simulink model "UTSG11111"  (R2016a)
settings: Solver=VariableStepAuto  StartTime=0.0  StopTime=10.0  RelTol=1e-3
values from neighbouring files (symbols this model uses):
  A_dw = 110.74    [zmienne.m]
  A_fs = 60.67    [zmienne.m]
  A_p = (PI * (D_i^2) * N) / (4 * 144)    (= 11.0984259136)    [zmienne.m]
  C_1 = 1 / sqrt(C_d)    [zmienne.m]
  C_m = 0.11    [zmienne.m]
  C_p1 = 1.39    [zmienne.m]
  C_p2 = 1.165    [zmienne.m]
  DENS_d = 50.32    [zmienne.m]
  DENS_dw = 47.66    [zmienne.m]
  DENS_s = 52.32    [zmienne.m]
  DENS_w = 45.710    (= 45.71)    [zmienne.m]
  G_1 = 65.2    [zmienne.m]
  G_2 = 1.0    (= 1)    [zmienne.m]
  G_v = 32.2    [zmienne.m]
  K1 = 3.5 * 10^-6    (= 3.5e-06)    [zmienne.m]
  K2 = -7.135 * 10^-4    (= -0.0007135)    [zmienne.m]
  K3 = 0.17    [zmienne.m]
  K4 = -0.2    [zmienne.m]
  K5 = 0.14    [zmienne.m]
  K7 = 2.37 * 10^-3    (= 0.00237)    [zmienne.m]
  L = 35.54    [zmienne.m]
  L_d = 35.54    [zmienne.m]
  L_dw0 = 9.63    [zmienne.m]
  L_r = 9.63    [zmienne.m]
  m0 = 0    [zmienne.m]
  M_d = DENS_d * A_d *L_d    (= 57227.9296)    [zmienne.m]
  M_m1 = (M_m * L_s10) / L    (= 5577.64460636)    [zmienne.m]
  M_m2 = M_m * (L_s20 / L)    (= 51851.8797758)    [zmienne.m]
  M_m3 = M_m2    (= 51851.8797758)    [zmienne.m]
  M_m4 = M_m1    (= 5577.64460636)    [zmienne.m]
  M_p1 = (M_p * L_s10) / L    (= 1751.07864275)    [zmienne.m]
  M_p2 = (M_p * L_s20) / L    (= 16278.6849414)    [zmienne.m]
  P_r2 = S_pm2 / L_s20    (= 687.386379167)    [zmienne.m]
  r0 = 0    [zmienne.m]
  S_ms1 = S_m * (L_s10 / L)    (= 2678.800154)    [zmienne.m]
  S_ms2 = S_m * (L_s20 / L)    (= 24903.1326539)    [zmienne.m]
  S_ms3 = S_ms2    (= 24903.1326539)    [zmienne.m]
  S_ms4 = S_ms1    (= 2678.800154)    [zmienne.m]
  S_pm1 = (S_ms1 * D_i) / D_o    (= 2372.65156497)    [zmienne.m]
  S_pm2 = (S_ms2 * D_i) / D_o    (= 22057.0603506)    [zmienne.m]
  S_pm3 = S_pm1    (= 2372.65156497)    [zmienne.m]
  S_pm4 = S_pm2    (= 22057.0603506)    [zmienne.m]
  tau = 5    [zmienne.m]
  tau_1 = 250    [zmienne.m]
  tau_2 = 120    [zmienne.m]
  tau_pi = M_pi / W_pi    (= 0.60183806901)    [zmienne.m]
  U_ms1 = 1 / (((1 / h_os) + (D_o * log(D_o/D_m))) / (24 * K_th))    [zmienne.m]
  U_ms2 = 1 / (((1 / h_ob) + (D_o * log(D_o/D_m))) / (24 * K_th))    [zmienne.m]
  U_pm = 1 / (((1 / h_i) + (D_i * log(D_m/D_i))) / (24 * K_th))    [zmienne.m]
  V_dr = 4398.706    [zmienne.m]
  V_r = 468.981    [zmienne.m]
  w0 = 0    [zmienne.m]
  W_fi0 = 1036.39    [zmienne.m]
  W_nv = 0.63    [zmienne.m]
  W_pi = 10941.6    [zmienne.m]
  X1 = 402.94    [zmienne.m]
  X2 = 0.018    [zmienne.m]
  X3 = 1.13096    [zmienne.m]
  X4 = 370.751    [zmienne.m]
  X5 = 850.04    [zmienne.m]
  X6 = -0.181289    [zmienne.m]
  Z_tv = 3.18    [zmienne.m]
undefined symbols (not defined in the file or in its folder): magnitude
(part 1 of 2)
settings Model: Creator=Użytkownik  LastModifiedBy=Użytkownik
settings GRTTargetCC: GeneratePreprocessorConditionals=Use local settings

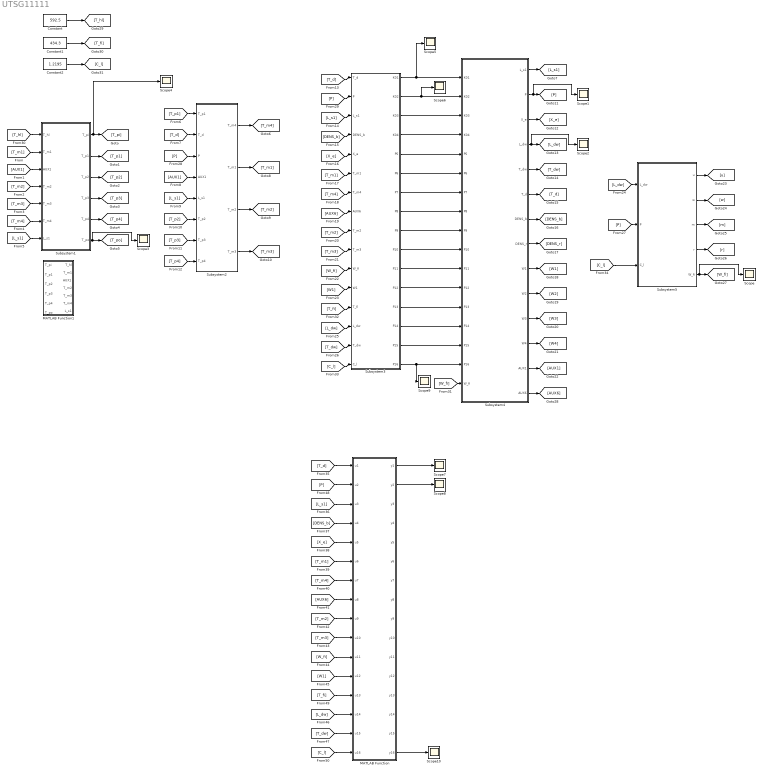
== system UTSG11111 ==
  Constant : Constant  Value=592.5
  Constant1 : Constant  Value=434.3
  Constant2 : Constant  Value=1.2195
  MATLAB Function : MATLAB Function  TreatAsAtomicUnit=on
  MATLAB Function1 : MATLAB Function  TreatAsAtomicUnit=on
  Scope{,1..10} (11 alike) : Scope
  Subsystem1 : Subsystem
  Subsystem2 : Subsystem
  Subsystem3 : Subsystem
  Subsystem4 : Subsystem
  Subsystem5 : Subsystem
  wires:
  Subsystem1/1(T_pi) -> Scope4/1, [T_pi]
  Subsystem1/2(T_p1) -> [T_p1]
  Subsystem1/3(T_p2) -> [T_p2]
  Subsystem1/4(T_p3) -> [T_p3]
  Subsystem1/5(T_p4) -> [T_p4]
  Subsystem1/6(T_po) -> Scope3/1, [T_po]
  Subsystem2/1(T_m4) -> [T_m4]
  Subsystem2/2(T_m1) -> [T_m1]
  Subsystem2/3(T_m2) -> [T_m2]
  Subsystem2/4(T_m3) -> [T_m3]
  Subsystem4/1(L_s1) -> [L_s1]
  Subsystem4/2(P) -> Scope1/1, [P]
  Subsystem4/3(X_e) -> [X_e]
  Subsystem4/4(L_dw) -> Scope2/1, [L_dw]
  Subsystem4/5(T_dw) -> [T_dw]
  Subsystem4/6(T_d) -> [T_d]
  Subsystem4/7(DENS_b) -> [DENS_b]
  Subsystem4/8(DENS_r) -> [DENS_r]
  Subsystem4/9(W1) -> [W1]
  Subsystem4/10(W2) -> [W2]
  Subsystem4/11(W3) -> [W3]
  Subsystem4/12(W4) -> [W4]
  Subsystem4/13(AUX1) -> [AUX1]
  [T_m1] -> Subsystem1/2(T_m1)
  [AUX1] -> Subsystem1/3(AUX1)
  [T_m2] -> Subsystem1/4(T_m2)
  [T_m3] -> Subsystem1/5(T_m3)
  [T_m4] -> Subsystem1/6(T_m4)
  [L_s1] -> Subsystem1/7(L_s1)
  Subsystem5/1(u) -> [u]
  Subsystem5/2(w) -> [w]
  Subsystem5/3(m) -> [m]
  Subsystem5/4(r) -> [r]
  Subsystem5/5(W_fi) -> Scope/1, [W_fi]
  [T_p1] -> Subsystem2/1(T_p1)
  [T_d] -> Subsystem2/2(T_d)
  [AUX1] -> Subsystem2/4(AUX1)
  [L_s1] -> Subsystem2/5(L_s1)
  [T_p2] -> Subsystem2/6(T_p2)
  [T_p3] -> Subsystem2/7(T_p3)
  [T_p4] -> Subsystem2/8(T_p4)
  [T_d] -> Subsystem3/1(T_d)
  [L_s1] -> Subsystem3/3(L_s1)
  [DENS_b] -> Subsystem3/4(DENS_b)
  [X_e] -> Subsystem3/5(X_e)
  [T_m1] -> Subsystem3/6(T_m1)
  [T_m4] -> Subsystem3/7(T_m4)
  [T_m2] -> Subsystem3/9(T_m2)
  [T_m3] -> Subsystem3/10(T_m3)
  [W_fi] -> Subsystem3/11(W_fi)
  [AUX6] -> Subsystem3/8(AUX6)
  Subsystem4/14(AUX6) -> [AUX6]
  [W1] -> Subsystem3/12(W1)
  [L_dw] -> Subsystem3/14(L_dw)
  [T_dw] -> Subsystem3/15(T_dw)
  [L_dw] -> Subsystem5/1(L_dw)
  [P] -> Subsystem5/2(P)
  [P] -> Subsystem2/3(P)
  [P] -> Subsystem3/2(P)
  [T_hl] -> Subsystem1/1(T_hl)
  [W_fi] -> Subsystem4/17(W_fi)
  [T_fi] -> Subsystem3/13(T_fi)
  [C_l] -> Subsystem3/16(C_l)
  [C_l] -> Subsystem5/3(C_l)
  Constant2/1 -> [C_l]
  Constant1/1 -> [T_fi]
  Constant/1 -> [T_hl]
  Subsystem3/1(K01) -> Scope5/1, Subsystem4/1(K01)
  Subsystem3/2(K02) -> Scope6/1, Subsystem4/2(K02)
  Subsystem3/3(K03) -> Subsystem4/3(K03)
  Subsystem3/4("K04 ") -> Subsystem4/4(K04)
  Subsystem3/5(P5) -> Subsystem4/5(P5)
  Subsystem3/6(P6) -> Subsystem4/6(P6)
  Subsystem3/7(P7) -> Subsystem4/7(P7)
  Subsystem3/8(P8) -> Subsystem4/8(P8)
  Subsystem3/9(P9) -> Subsystem4/9(P9)
  Subsystem3/10(P10) -> Subsystem4/10(P10)
  Subsystem3/11(P11) -> Subsystem4/11(P11)
  Subsystem3/12(P12) -> Subsystem4/12(P12)
  Subsystem3/13(P13) -> Subsystem4/13(P13)
  Subsystem3/14(P14) -> Subsystem4/14(P14)
  Subsystem3/15(P15) -> Subsystem4/15(P15)
  Subsystem3/16(P16) -> Scope9/1, Subsystem4/16(P16)
  [T_d] -> MATLAB Function/1(u1)
  [P] -> MATLAB Function/2(u2)
  [L_s1] -> MATLAB Function/3(u3)
  [DENS_b] -> MATLAB Function/4(u4)
  [X_e] -> MATLAB Function/5(u5)
  [T_m1] -> MATLAB Function/6(u6)
  [T_m4] -> MATLAB Function/7(u7)
  [AUX6] -> MATLAB Function/8(u8)
  [T_m2] -> MATLAB Function/9(u9)
  [T_m3] -> MATLAB Function/10(u10)
  [W_fi] -> MATLAB Function/11(u11)
  [W1] -> MATLAB Function/12(u12)
  [T_fi] -> MATLAB Function/13(u13)
  [L_dw] -> MATLAB Function/14(u14)
  [T_dw] -> MATLAB Function/15(u15)
  [C_l] -> MATLAB Function/16(u16)
  MATLAB Function/1(y1) -> Scope7/1
  MATLAB Function/2(y2) -> Scope8/1
  MATLAB Function/16(y16) -> Scope10/1

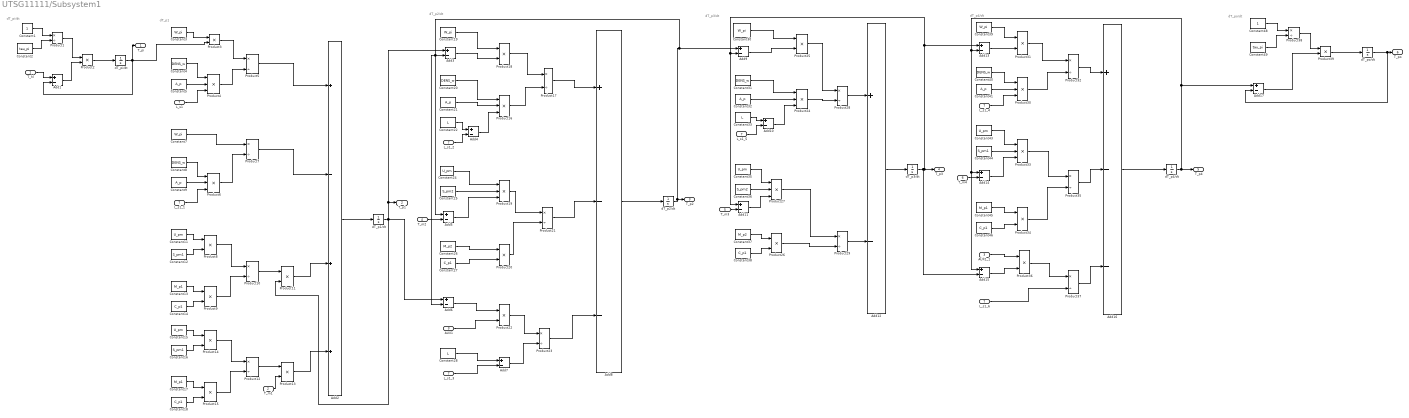
== system UTSG11111/Subsystem1 ==
  note: dT_po/dt
  note: dT_p4/dt
  note: dT_p3/dt
  note: dT_p2/dt
  note: dT_p1
  note: dT_pi/dt
  T_hl : Inport
  T_m1 : Inport  Port=2
  AUX1 : Inport  Port=3
  T_m2 : Inport  Port=4
  T_m3 : Inport  Port=5
  T_m4 : Inport  Port=6
  L_s1 : Inport  Port=7
  AUX1_1 : InportShadow  Port=3
  Add{1,3..7,9..15,17} (14 alike) : Sum  Inputs=+-
  Add16 : Sum  Inputs=+--
  Add2 : Sum  Inputs=+-++
  Add8 : Sum  Inputs=+--
  Constant1 : Constant
  Constant{11,15,24,35,43} (5 alike) : Constant  Value=U_pm
  Constant12 : Constant  Value=S_pm1
  Constant13 : Constant  Value=M_p1
  Constant{14,18,27,38,46} (5 alike) : Constant  Value=C_p1
  Constant16 : Constant  Value=S_pm1
  Constant17 : Constant  Value=M_p1
  Constant{3,7,19,30,39} (5 alike) : Constant  Value=W_pi
  Constant2 : Constant  Value=tau_pi
  Constant{4,8,20,31,40} (5 alike) : Constant  Value=DENS_w
  Constant{5,9,21,32,41} (5 alike) : Constant  Value=A_p
  Constant22 : Constant  Value=L
  Constant25 : Constant  Value=S_pm2
  Constant26 : Constant  Value=M_p2
  Constant28 : Constant  Value=L
  Constant33 : Constant  Value=L
  Constant36 : Constant  Value=S_pm2
  Constant37 : Constant  Value=M_p2
  Constant44 : Constant  Value=S_pm1
  Constant45 : Constant  Value=M_p1
  Constant48 : Constant
  Constant49 : Constant  Value=tau_pi
  L_s1_{1..6} (6 alike) : InportShadow  Port=7
  Product{1,5,7,10,12,17,21,23,28..29,32,35,37..38} (14 alike) : Product  Inputs=*/
  Product{2..3,8..9,11,13..15,18,20,22,25..26,31,34,36,39} (17 alike) : Product
  Product{4,6,16,19,24,27,30,33} (8 alike) : Product  Inputs=3
  dT_p1/dt : Integrator  InitialCondition=587.36
  dT_p2/dt : Integrator  InitialCondition=557.4
  dT_p3/dt : Integrator  InitialCondition=542.5
  dT_p4/dt : Integrator  InitialCondition=539.5
  dT_pi/dt : Integrator  InitialCondition=592.5
  dT_po/dt : Integrator  InitialCondition=539.5
  T_pi : Outport
  T_p1 : Outport  Port=2
  T_p2 : Outport  Port=3
  T_p3 : Outport  Port=4
  T_p4 : Outport  Port=5
  T_po : Outport  Port=6
  wires:
  Constant1/1 -> Product1/1
  Constant2/1 -> Product1/2
  T_hl/1 -> Add1/1
  Product1/1 -> Product2/1
  Add1/1 -> Product2/2
  Product2/1 -> dT_pi/dt/1
  dT_pi/dt/1 -> T_pi/1, Product3/2, Add1/2
  Constant3/1 -> Product3/1
  Constant4/1 -> Product4/1
  Constant5/1 -> Product4/2
  L_s1/1 -> Product4/3
  Product3/1 -> Product5/1
  Product4/1 -> Product5/2
  Constant8/1 -> Product6/1
  Constant9/1 -> Product6/2
  L_s1_1/1 -> Product6/3
  Constant7/1 -> Product7/1
  Product6/1 -> Product7/2
  Constant11/1 -> Product8/1
  Constant12/1 -> Product8/2
  Constant13/1 -> Product9/1
  Constant14/1 -> Product9/2
  Product8/1 -> Product10/1
  Product9/1 -> Product10/2
  Product10/1 -> Product11/1
  Constant15/1 -> Product14/1
  Constant16/1 -> Product14/2
  Constant17/1 -> Product15/1
  Constant18/1 -> Product15/2
  Product14/1 -> Product12/1
  Product15/1 -> Product12/2
  Product12/1 -> Product13/1
  T_m1/1 -> Product13/2
  Product5/1 -> Add2/1
  Product7/1 -> Add2/2
  Product11/1 -> Add2/3
  Product13/1 -> Add2/4
  dT_p1/dt/1 -> Add6/1, Product11/2, T_p1/1, Add3/1
  Add2/1 -> dT_p1/dt/1
  Constant22/1 -> Add4/1
  L_s1_2/1 -> Add4/2
  Constant20/1 -> Product16/1
  Constant21/1 -> Product16/2
  Add4/1 -> Product16/3
  Constant19/1 -> Product18/1
  Add3/1 -> Product18/2
  Product18/1 -> Product17/1
  Product16/1 -> Product17/2
  Add5/1 -> Product19/3
  Constant25/1 -> Product19/2
  Constant24/1 -> Product19/1
  Constant26/1 -> Product20/1
  Constant27/1 -> Product20/2
  Product19/1 -> Product21/1
  Product20/1 -> Product21/2
  dT_p2/dt/1 -> T_p2/1, Add5/1, Add3/2, Add6/2, Add9/1
  Add6/1 -> Product22/1
  AUX1/1 -> Product22/2
  Constant28/1 -> Add7/1
  L_s1_3/1 -> Add7/2
  Product22/1 -> Product23/1
  Add7/1 -> Product23/2
  Add8/1 -> dT_p2/dt/1
  Product17/1 -> Add8/1
  Product21/1 -> Add8/2
  Product23/1 -> Add8/3
  Constant33/1 -> Add10/1
  L_s1_5/1 -> Add10/2
  Constant31/1 -> Product24/1
  Constant32/1 -> Product24/2
  Add10/1 -> Product24/3
  Constant30/1 -> Product25/1
  Add9/1 -> Product25/2
  dT_p3/dt/1 -> T_p3/1, Add11/1, Add9/2, Add13/1, Add15/2
  Constant37/1 -> Product26/1
  Constant38/1 -> Product26/2
  Constant35/1 -> Product27/1
  Constant36/1 -> Product27/2
  Add11/1 -> Product27/3
  T_m2/1 -> Add5/2
  T_m3/1 -> Add11/2
  Add12/1 -> dT_p3/dt/1
  Product28/1 -> Add12/1
  Product25/1 -> Product28/1
  Product24/1 -> Product28/2
  Product29/1 -> Add12/2
  Product27/1 -> Product29/1
  Product26/1 -> Product29/2
  dT_p4/dt/1 -> T_p4/1, Add17/1, Add15/1, Add14/1, Add13/2
  Constant41/1 -> Product30/2
  Constant40/1 -> Product30/1
  L_s1_4/1 -> Product30/3
  Constant39/1 -> Product31/1
  Add13/1 -> Product31/2
  Product31/1 -> Product32/1
  Product30/1 -> Product32/2
  T_m4/1 -> Add14/2
  Constant43/1 -> Product33/1
  Constant44/1 -> Product33/2
  Add14/1 -> Product33/3
  Constant45/1 -> Product34/1
  Constant46/1 -> Product34/2
  Product33/1 -> Product35/1
  Product34/1 -> Product35/2
  AUX1_1/1 -> Product36/1
  Add15/1 -> Product36/2
  Product36/1 -> Product37/1
  L_s1_6/1 -> Product37/2
  Add16/1 -> dT_p4/dt/1
  Product32/1 -> Add16/1
  Product35/1 -> Add16/2
  Product37/1 -> Add16/3
  Constant48/1 -> Product38/1
  Constant49/1 -> Product38/2
  dT_po/dt/1 -> Add17/2, T_po/1
  Product38/1 -> Product39/1
  Add17/1 -> Product39/2
  Product39/1 -> dT_po/dt/1

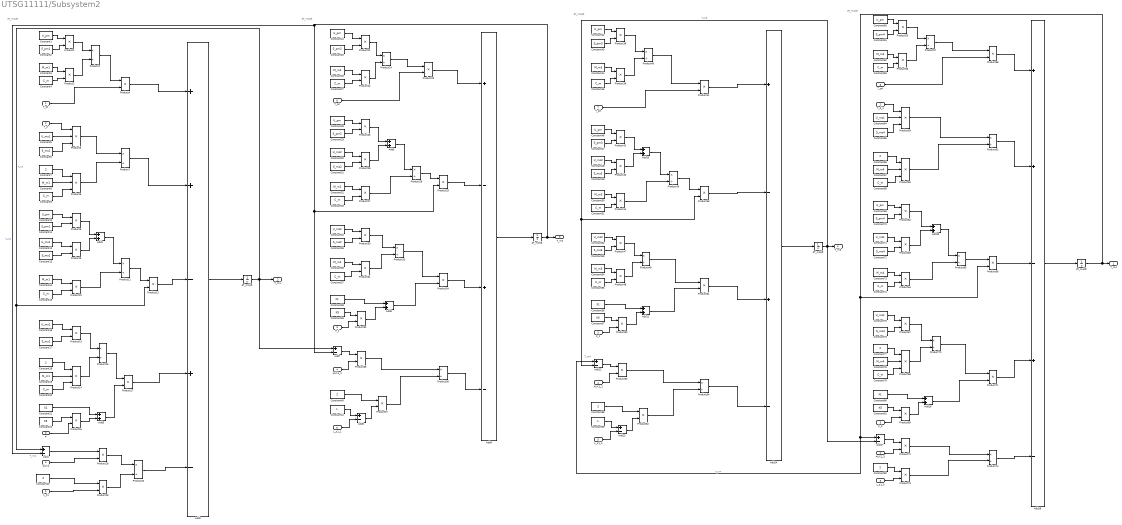
== system UTSG11111/Subsystem2 ==
  note: dT_m4/dt
  note: dT_m3/dt
  note: T_m4
  note: dT_m2/dt
  note: dT_m1/dt
  note: T_m2
  T_p1 : Inport
  T_d : Inport  Port=2
  P : Inport  Port=3
  AUX1 : Inport  Port=4
  L_s1 : Inport  Port=5
  T_p2 : Inport  Port=6
  T_p3 : Inport  Port=7
  T_p4 : Inport  Port=8
  AUX1_1 : InportShadow  Port=4
  AUX1_2 : InportShadow  Port=4
  AUX1_3 : InportShadow  Port=4
  Add{1,3,5..6,10..11,15..16} (8 alike) : Sum
  Add{4,7..8,12..13,17} (6 alike) : Sum  Inputs=+-
  Add14 : Sum  Inputs=+-+-
  Add18 : Sum  Inputs=++-+-
  Add2 : Sum  Inputs=++-+-
  Add9 : Sum  Inputs=+-+-
  Constant{1,10,24,28,42,46,60,69} (8 alike) : Constant  Value=U_pm
  Constant11 : Constant  Value=S_pm1
  Constant{5,12,16,64,71,75} (6 alike) : Constant  Value=U_ms1
  Constant13 : Constant  Value=S_ms1
  Constant{3,8,14,19} (4 alike) : Constant  Value=M_m1
  Constant{4,9,15,20,27,33,37,45,51,55,63,68,74,79} (14 alike) : Constant  Value=C_m
  Constant17 : Constant  Value=S_ms1
  Constant{7,18,23,40,58,66,77,82} (8 alike) : Constant  Value=2
  Constant2 : Constant  Value=S_pm1
  Constant{21,38,56,80} (4 alike) : Constant  Value=X1
  Constant{22,39,57,81} (4 alike) : Constant  Value=K5
  Constant25 : Constant  Value=S_pm2
  Constant26 : Constant  Value=M_m2
  Constant29 : Constant  Value=S_pm2
  Constant{30,34,48,52} (4 alike) : Constant  Value=U_ms2
  Constant31 : Constant  Value=S_ms2
  Constant32 : Constant  Value=M_m2
  Constant35 : Constant  Value=S_ms2
  Constant36 : Constant  Value=M_m2
  Constant41 : Constant  Value=L
  Constant43 : Constant  Value=S_pm3
  Constant44 : Constant  Value=M_m3
  Constant47 : Constant  Value=S_pm3
  Constant49 : Constant  Value=S_ms3
  Constant50 : Constant  Value=M_m3
  Constant53 : Constant  Value=S_ms3
  Constant54 : Constant  Value=M_m3
  Constant59 : Constant  Value=L
  Constant6 : Constant  Value=S_ms1
  Constant61 : Constant  Value=S_pm4
  Constant{62,67,73,78} (4 alike) : Constant  Value=M_m4
  Constant65 : Constant  Value=S_ms4
  Constant70 : Constant  Value=S_pm4
  Constant72 : Constant  Value=S_ms4
  Constant76 : Constant  Value=S_ms4
  L_s1_1 : InportShadow  Port=5
  L_s1_2 : InportShadow  Port=5
  L_s1_3 : InportShadow  Port=5
  P_1 : InportShadow  Port=3
  P_2 : InportShadow  Port=3
  P_3 : InportShadow  Port=3
  Product{1..2,4,8..10,12..13,15,17..19,21..23,25..27,29..32,34..35,37..39,41..44,46..48,50..53,55..56,58,62..64,66..67,69,71..73} (50 alike) : Product
  Product{3,7,11,16,20,24,28,33,36,40,45,49,54,57,61,65,70,74} (18 alike) : Product  Inputs=*/
  Product{5..6,14,59..60,68} (6 alike) : Product  Inputs=3
  T_d_1 : InportShadow  Port=2
  dT_m1/dt : Integrator  InitialCondition=553.49
  dT_m2/dt : Integrator  InitialCondition=536.129
  dT_m3/dt : Integrator  InitialCondition=529.38
  dT_m4/dt : Integrator  InitialCondition=527.38
  T_m4 : Outport
  T_m1 : Outport  Port=2
  T_m2 : Outport  Port=3
  T_m3 : Outport  Port=4
  wires:
  Constant1/1 -> Product1/1
  Constant2/1 -> Product1/2
  Constant3/1 -> Product2/1
  Constant4/1 -> Product2/2
  Product1/1 -> Product3/1
  Product2/1 -> Product3/2
  T_p1/1 -> Product4/2
  Product3/1 -> Product4/1
  T_d/1 -> Product5/1
  Constant5/1 -> Product5/2
  Constant6/1 -> Product5/3
  Constant8/1 -> Product6/2
  Constant7/1 -> Product6/1
  Constant9/1 -> Product6/3
  Product5/1 -> Product7/1
  Product6/1 -> Product7/2
  Constant10/1 -> Product8/1
  Constant11/1 -> Product8/2
  Constant12/1 -> Product9/1
  Constant13/1 -> Product9/2
  Product8/1 -> Add1/1
  Product9/1 -> Add1/2
  Constant14/1 -> Product10/1
  Constant15/1 -> Product10/2
  Add1/1 -> Product11/1
  Product10/1 -> Product11/2
  Product11/1 -> Product12/1
  dT_m1/dt/1 -> Add7/1, T_m1/1, Add4/1, Product12/2  "T_m1"
  Constant16/1 -> Product13/1
  Constant17/1 -> Product13/2
  Constant19/1 -> Product14/2
  Constant18/1 -> Product14/1
  Constant20/1 -> Product14/3
  Constant21/1 -> Add3/1
  Constant22/1 -> Product15/1
  P/1 -> Product15/2
  Product13/1 -> Product16/1
  Product14/1 -> Product16/2
  Product16/1 -> Product17/1
  Add3/1 -> Product17/2
  Product4/1 -> Add2/1
  Product7/1 -> Add2/2
  Product12/1 -> Add2/3
  Product17/1 -> Add2/4
  Add4/1 -> Product18/1
  AUX1/1 -> Product18/2
  Constant23/1 -> Product19/1
  L_s1/1 -> Product19/2
  Add2/1 -> dT_m1/dt/1
  Product18/1 -> Product20/1
  Product19/1 -> Product20/2
  Product20/1 -> Add2/5
  Constant24/1 -> Product21/1
  Constant25/1 -> Product21/2
  Constant26/1 -> Product22/1
  Constant27/1 -> Product22/2
  T_p2/1 -> Product23/2
  Product21/1 -> Product24/1
  Product22/1 -> Product24/2
  Product24/1 -> Product23/1
  Constant30/1 -> Product26/1
  Constant31/1 -> Product26/2
  Constant28/1 -> Product25/1
  Constant29/1 -> Product25/2
  Constant32/1 -> Product27/1
  Constant33/1 -> Product27/2
  Product25/1 -> Add5/1
  Product26/1 -> Add5/2
  Add5/1 -> Product28/1
  Product27/1 -> Product28/2
  Product28/1 -> Product29/1
  dT_m2/dt/1 -> T_m2/1, Add4/2, Add7/2, Product29/2  "T_m2"
  Constant34/1 -> Product30/1
  Constant35/1 -> Product30/2
  Constant36/1 -> Product31/1
  Constant37/1 -> Product31/2
  Constant39/1 -> Product32/1
  P_1/1 -> Product32/2
  Constant38/1 -> Add6/1
  Product32/1 -> Add6/2
  Product15/1 -> Add3/2
  Product30/1 -> Product33/1
  Product31/1 -> Product33/2
  Product33/1 -> Product34/1
  Add6/1 -> Product34/2
  Add7/1 -> Product35/1
  AUX1_1/1 -> Product35/2
  Product35/1 -> Product36/1
  Constant41/1 -> Add8/1
  L_s1_1/1 -> Add8/2
  Constant40/1 -> Product37/1
  Add8/1 -> Product37/2
  Product37/1 -> Product36/2
  Product23/1 -> Add9/1
  Product29/1 -> Add9/2
  Product34/1 -> Add9/3
  Product36/1 -> Add9/4
  Add9/1 -> dT_m2/dt/1
  Constant42/1 -> Product38/1
  Constant43/1 -> Product38/2
  Constant44/1 -> Product39/1
  Constant45/1 -> Product39/2
  Product38/1 -> Product40/1
  Product39/1 -> Product40/2
  Product40/1 -> Product41/1
  T_p3/1 -> Product41/2
  Constant46/1 -> Product42/1
  Constant47/1 -> Product42/2
  Constant48/1 -> Product43/1
  Constant49/1 -> Product43/2
  Product42/1 -> Add10/1
  Product43/1 -> Add10/2
  Constant50/1 -> Product44/1
  Constant51/1 -> Product44/2
  Add10/1 -> Product45/1
  Product44/1 -> Product45/2
  Product45/1 -> Product46/1
  dT_m3/dt/1 -> Add17/2, Add12/2, Product46/2, T_m3/1  "T_m3"
  Constant52/1 -> Product47/1
  Constant53/1 -> Product47/2
  Constant54/1 -> Product48/1
  Constant55/1 -> Product48/2
  Product47/1 -> Product49/1
  Product48/1 -> Product49/2
  Constant57/1 -> Product50/1
  P_2/1 -> Product50/2
  Constant56/1 -> Add11/1
  Product50/1 -> Add11/2
  Product49/1 -> Product51/1
  Add11/1 -> Product51/2
  Constant59/1 -> Add13/1
  L_s1_2/1 -> Add13/2
  Constant58/1 -> Product52/1
  Add13/1 -> Product52/2
  Add12/1 -> Product53/1
  AUX1_2/1 -> Product53/2
  Product53/1 -> Product54/1
  Product52/1 -> Product54/2
  Product41/1 -> Add14/1
  Product46/1 -> Add14/2
  Product51/1 -> Add14/3
  Product54/1 -> Add14/4
  Add14/1 -> dT_m3/dt/1
  Constant60/1 -> Product55/1
  Constant61/1 -> Product55/2
  Constant62/1 -> Product56/1
  Constant63/1 -> Product56/2
  Product55/1 -> Product57/1
  Product56/1 -> Product57/2
  T_p4/1 -> Product58/2
  Product57/1 -> Product58/1
  T_d_1/1 -> Product59/1
  Constant64/1 -> Product59/2
  Constant65/1 -> Product59/3
  Constant66/1 -> Product60/1
  Constant67/1 -> Product60/2
  Constant68/1 -> Product60/3
  Product59/1 -> Product61/1
  Product60/1 -> Product61/2
  Constant69/1 -> Product62/1
  Constant70/1 -> Product62/2
  Constant71/1 -> Product63/1
  Constant72/1 -> Product63/2
  Constant73/1 -> Product64/1
  Constant74/1 -> Product64/2
  Product62/1 -> Add15/1
  Product63/1 -> Add15/2
  Add15/1 -> Product65/1
  Product64/1 -> Product65/2
  dT_m4/dt/1 -> T_m4/1, Product66/2, Add17/1, Add12/1  "T_m4"
  Product65/1 -> Product66/1
  Constant75/1 -> Product67/1
  Constant76/1 -> Product67/2
  Constant77/1 -> Product68/1
  Constant78/1 -> Product68/2
  Constant79/1 -> Product68/3
  Constant81/1 -> Product69/1
  P_3/1 -> Product69/2
  Constant80/1 -> Add16/1
  Product69/1 -> Add16/2
  Product67/1 -> Product70/1
  Product68/1 -> Product70/2
  Product70/1 -> Product71/1
  Add16/1 -> Product71/2
  Add17/1 -> Product72/1
  AUX1_3/1 -> Product72/2
  Constant82/1 -> Product73/1
  L_s1_3/1 -> Product73/2
  Product72/1 -> Product74/1
  Product73/1 -> Product74/2
  Product58/1 -> Add18/1
  Product61/1 -> Add18/2
  Product66/1 -> Add18/3
  Product71/1 -> Add18/4
  Product74/1 -> Add18/5
  Add18/1 -> dT_m4/dt/1

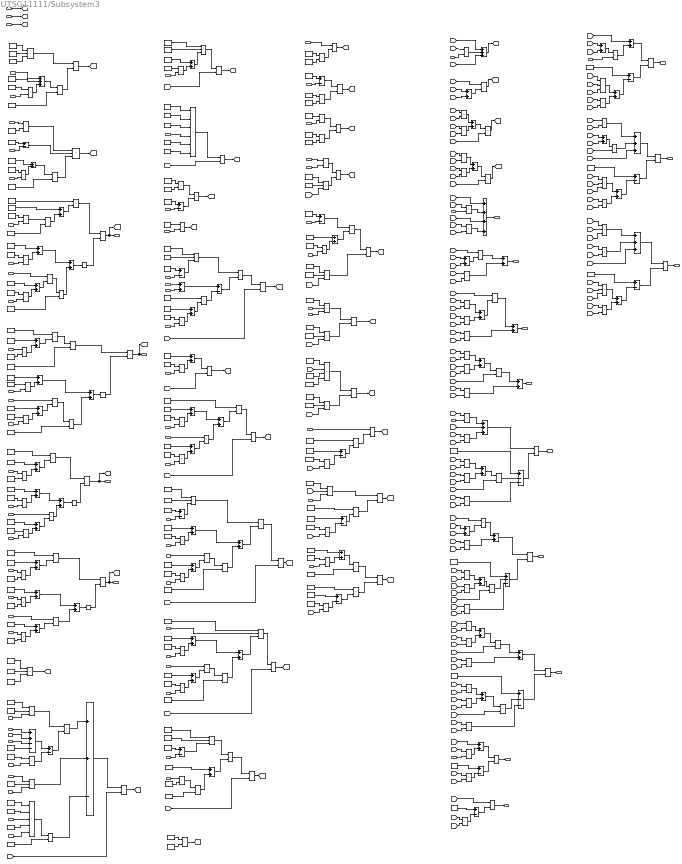
== system UTSG11111/Subsystem3 ==
  note: P16
  note: P15
  note: P14
  note: P13
  note: P12
  note: P11
  note: P10
  note: P9
  note: P8
  note: P7
  note: P6
  note: P5
  note: P4
  note: P3
  note: P2
  note: P1
  note: K027
  note: K026
  note: K025
  note: K024
  note: K023
  note: K022
  note: K021
  note: K020
  note: K019
  note: K018
  note: K017
  note: K016
  note: K015
  note: K014
  note: K013
  note: K012
  note: K011
  note: K010
  note: K09
  note: K08
  note: K07
  note: K06
  note: K05
  note: K04
  note: K03
  note: K02
  note: K01
  note: DEN2
  note: DEN1
  T_d : Inport
  P : Inport  Port=2
  L_s1 : Inport  Port=3
  DENS_b : Inport  Port=4
  X_e : Inport  Port=5
  T_m1 : Inport  Port=6
  T_m4 : Inport  Port=7
  AUX6 : Inport  Port=8
  T_m2 : Inport  Port=9
  T_m3 : Inport  Port=10
  W_fi : Inport  Port=11
  W1 : Inport  Port=12
  T_fi : Inport  Port=13
  L_dw : Inport  Port=14
  T_dw : Inport  Port=15
  C_l : Inport  Port=16
  Add1 : Sum  Inputs=+++
  Add{3..19,23,26..27,29..34,36..39,42,45,48,51,53,56..62,64,66..68,70..72,74,77..79,81,83,85} (56 alike) : Sum
  Add{2,21,24..25,28,35,41,43..44,46..47,49,75..76,80,84,86} (17 alike) : Sum  Inputs=+-
  Add20 : Sum  Inputs=++--
  Add22 : Sum  Inputs=++-
  Add50 : Sum  Inputs=+++
  Add52 : Sum  Inputs=++++
  Add63 : Sum  Inputs=3
  Add65 : Sum  Inputs=+--
  Add69 : Sum  Inputs=+--
  Add73 : Sum  Inputs=+--
  Add82 : Sum  Inputs=3
  Add87 : Sum  Inputs=3
  Constant{1,8,46,54,62,67,69,84,91,98} (10 alike) : Constant  Value=A_fs
  Constant{10,80,88,94} (4 alike) : Constant  Value=X5
  Constant{77,79,87,93,100} (5 alike) : Constant  Value=K3
  Constant{11,81,89,95,101} (5 alike) : Constant  Value=K4
  Constant{6,12,14,19,24,28,57,73,90,96,102} (11 alike) : Constant  Value=2
  Constant{20..21,30,37,44,60..61,66,82..83,103..104,111,127,134,139} (16 alike) : Constant  Value=-1
  Constant105 : Constant  Value=V_r
  Constant{106,109,112,115,121,124,128,130,137,143,147,151} (12 alike) : Constant  Value=A_dw
  Constant{107,110,113,116,122,125,129,131} (8 alike) : Constant  Value=DENS_dw
  Constant{108,118,152..159} (10 alike) : Constant
  Constant{4,50,58,74,119} (5 alike) : Constant  Value=X1
  Constant{5,51,59,65,75,120} (6 alike) : Constant  Value=K5
  Constant{13,18,23,27,32,36,39,43} (8 alike) : Constant  Value=K2
  Constant{135,141,146,148} (4 alike) : Constant  Value=K7
  Constant136 : Constant  Value=V_dr
  Constant142 : Constant  Value=V_dr
  Constant145 : Constant  Value=X6
  Constant149 : Constant  Value=V_dr
  Constant{15,29,33,40} (4 alike) : Constant  Value=X2
  Constant{7,16,25,31,34,41} (6 alike) : Constant  Value=K1
  Constant{17,22,26,35,38,42} (6 alike) : Constant  Value=X3
  Constant{2,45,55,63} (4 alike) : Constant  Value=DENS_s
  Constant{3,49,53,56,64} (5 alike) : Constant  Value=C_p2
  Constant47 : Constant  Value=U_ms1
  Constant48 : Constant  Value=P_r2
  Constant{9,68,72,85,99} (5 alike) : Constant  Value=L
  Constant70 : Constant  Value=U_ms2
  Constant71 : Constant  Value=P_r2
  Constant{76,78,86,92} (4 alike) : Constant  Value=X4
  DENS_b_1 : InportShadow  Port=4
  DENS_b_2 : InportShadow  Port=4
  L_s1_{1..7} (7 alike) : InportShadow  Port=3
  Math Function{,1..3} (4 alike) : Math  Operator=magnitude^2  SaturateOnIntegerOverflow=on
  P_{1..24} (24 alike) : InportShadow  Port=2
  Product{1,8,41..42,45,50,57,72,81,85,97,100,103..104,107,114,168,173,176,178} (20 alike) : Product  Inputs=3
  Product{3,7,10,15..17,23,33,40,47..48,51,53,61,63,68,73,75,79,82,84,87,90,92,95,98,102,105,108,111,115,120,145,152,161,164,166,170,175,180} (40 alike) : Product  Inputs=*/
  Product{2,4..6,9,11..14,18..22,24..31,34..38,43..44,49,54..56,58..60,62,64..67,69..71,74,76..78,83,86,88..89,91,93..94,96,99,101,109..110,112..113,116..119,121..144,146..151,153..160,162..163,165,167,169,171..172,174,177,179} (114 alike) : Product
  Product106 : Product  Inputs=4
  Product46 : Product  Inputs=5
  Product52 : Product  Inputs=6
  T_d_1 : InportShadow
  T_d_2 : InportShadow
  T_d_3 : InportShadow
  W1_{1..7} (7 alike) : InportShadow  Port=12
  W_fi_1 : InportShadow  Port=11
  X_e_{1..12} (12 alike) : InportShadow  Port=5
  K01 : Outport
  K02 : Outport  Port=2
  K03 : Outport  Port=3
  "K04 " : Outport  Port=4
  P5 : Outport  Port=5
  P6 : Outport  Port=6
  P7 : Outport  Port=7
  P8 : Outport  Port=8
  P9 : Outport  Port=9
  P10 : Outport  Port=10
  P11 : Outport  Port=11
  P12 : Outport  Port=12
  P13 : Outport  Port=13
  P14 : Outport  Port=14
  P15 : Outport  Port=15
  P16 : Outport  Port=16
  wires:
  Constant1/1 -> Product1/1
  Constant2/1 -> Product1/2
  Constant3/1 -> Product1/3
  Constant5/1 -> Product2/1
  P/1 -> Product2/2
  T_d/1 -> Add1/1
  Constant4/1 -> Add1/2
  Product2/1 -> Add1/3
  Add1/1 -> Product3/1
  Constant6/1 -> Product3/2
  Product1/1 -> Product4/1
  Product3/1 -> Product4/2
  Product4/1 -> [DEN1]
  DENS_b/1 -> Product5/1
  Constant8/1 -> Product5/2
  Constant9/1 -> Add2/1
  L_s1/1 -> Add2/2
  Constant12/1 -> Product7/2
  Product7/1 -> Product8/3
  Add2/1 -> Product8/2
  Constant11/1 -> Product6/1
  P_1/1 -> Product6/2
  Product6/1 -> Add3/2
  Constant10/1 -> Add3/1
  Add3/1 -> Product7/1
  Product5/1 -> Product8/1
  Product8/1 -> [DEN2]
  Constant13/1 -> Product9/1
  X_e/1 -> Product9/2
  Constant14/1 -> Product10/2
  Product9/1 -> Product10/1
  Constant7/1 -> Add4/1
  Product10/1 -> Add4/2
  Constant20/1 -> Product11/1
  Add4/1 -> Product11/2
  Constant16/1 -> Product12/1
  P_2/1 -> Product12/2
  Constant15/1 -> Add5/1
  Product12/1 -> Add5/2
  Constant18/1 -> Product13/1
  P_3/1 -> Product13/2
  Constant17/1 -> Add6/1
  Product13/1 -> Add6/2
  X_e_1/1 -> Product14/1
  Add6/1 -> Product14/2
  Product14/1 -> Product15/1
  Constant19/1 -> Product15/2
  Product15/1 -> Add7/2
  Add5/1 -> Add7/1
  Product11/1 -> Product17/1
  Math Function/1 -> Product17/2
  Product17/1 -> [K01], K01/1
  P_4/1 -> Product18/1
  Constant23/1 -> Product18/2
  Constant22/1 -> Add8/1
  Product18/1 -> Add8/2
  Constant21/1 -> Product19/1
  Add8/1 -> Product19/2
  Constant25/1 -> Product20/1
  P_5/1 -> Product20/2
  Product20/1 -> Add9/2
  Constant29/1 -> Add9/1
  Constant27/1 -> Product21/1
  P_6/1 -> Product21/2
  Constant26/1 -> Add10/1
  Product21/1 -> Add10/2
  X_e_2/1 -> Product22/1
  Add10/1 -> Product22/2
  Product22/1 -> Product23/1
  Constant28/1 -> Product23/2
  Add9/1 -> Add11/1
  Product23/1 -> Add11/2
  Math Function1/1 -> Product25/2
  Product25/1 -> [K02], K02/1
  Constant32/1 -> Product27/2
  X_e_3/1 -> Product27/1
  Constant31/1 -> Add12/1
  Product27/1 -> Add12/2
  Constant30/1 -> Product28/1
  Add12/1 -> Product28/2
  Constant34/1 -> Product29/1
  P_7/1 -> Product29/2
  Constant33/1 -> Add13/1
  Product29/1 -> Add13/2
  Constant36/1 -> Product30/1
  P_8/1 -> Product30/2
  Product30/1 -> Add14/2
  Constant35/1 -> Add14/1
  Add14/1 -> Product31/2
  X_e_4/1 -> Product31/1
  Product31/1 -> Add15/2
  Add13/1 -> Add15/1
  Product28/1 -> Product33/1
  Math Function2/1 -> Product33/2
  Product33/1 -> [K03], K03/1
  P_9/1 -> Product34/1
  Constant39/1 -> Product34/2
  Constant38/1 -> Add16/1
  Product34/1 -> Add16/2
  Constant37/1 -> Product35/1
  Add16/1 -> Product35/2
  P_10/1 -> Product36/1
  Constant41/1 -> Product36/2
  Constant40/1 -> Add17/1
  Product36/1 -> Add17/2
  P_11/1 -> Product37/1
  Constant43/1 -> Product37/2
  Constant42/1 -> Add18/1
  Product37/1 -> Add18/2
  X_e_5/1 -> Product38/1
  Add18/1 -> Product38/2
  Add17/1 -> Add19/1
  Product38/1 -> Add19/2
  Product35/1 -> Product40/1
  Math Function3/1 -> Product40/2
  Product40/1 -> [K04], "K04 "/1
  Constant44/1 -> Product41/1
  Constant45/1 -> Product41/2
  Constant46/1 -> Product41/3
  Product41/1 -> [K05]
  Constant47/1 -> Product42/1
  Constant48/1 -> Product42/2
  L_s1_2/1 -> Product42/3
  T_m1/1 -> Add20/1
  T_m4/1 -> Add20/2
  T_d_1/1 -> Add20/3
  Constant50/1 -> Add20/4
  Constant51/1 -> Product43/1
  P_12/1 -> Product43/2
  Add20/1 -> Add21/1
  Product43/1 -> Add21/2
  Product42/1 -> Product44/1
  Add21/1 -> Product44/2
  W1_7/1 -> Product45/1
  Constant53/1 -> Product45/2
  T_d_2/1 -> Product45/3
  Constant54/1 -> Product46/1
  Constant55/1 -> Product46/2
  L_s1_1/1 -> Product46/3
  Constant56/1 -> Product46/4
  AUX6/1 -> Product46/5
  Constant57/1 -> Product48/2
  Product46/1 -> Product48/1
  Product44/1 -> Add22/1
  Product45/1 -> Add22/2
  Product48/1 -> Add22/3
  Add22/1 -> Product47/1
  [DEN1] -> Product47/2
  Product47/1 -> [K06]
  Constant59/1 -> Product49/1
  P_13/1 -> Product49/2
  Constant58/1 -> Add23/1
  Product49/1 -> Add23/2
  Add23/1 -> Product50/3
  Constant49/1 -> Product50/2
  Constant60/1 -> Product50/1
  Product50/1 -> Product51/1
  [DEN1] -> Product51/2
  Product51/1 -> [K07]
  Constant61/1 -> Product52/1
  Constant62/1 -> Product52/2
  Constant63/1 -> Product52/3
  L_s1_3/1 -> Product52/4
  Constant64/1 -> Product52/5
  Constant65/1 -> Product52/6
  Product52/1 -> Product53/1
  [DEN1] -> Product53/2
  Product53/1 -> [K08]
  Constant66/1 -> Product54/1
  Constant67/1 -> Product54/2
  Constant68/1 -> Add24/1
  L_s1_4/1 -> Add24/2
  Product54/1 -> Product55/1
  Add24/1 -> Product55/2
  Product55/1 -> [K09]
  Constant69/1 -> Product56/1
  DENS_b_1/1 -> Product56/2
  Product56/1 -> [K010]
  Constant72/1 -> Add25/1
  L_s1_5/1 -> Add25/2
  Constant70/1 -> Product57/1
  Constant71/1 -> Product57/2
  Add25/1 -> Product57/3
  Constant75/1 -> Product58/1
  P_14/1 -> Product58/2
  T_m2/1 -> Add26/1
  T_m3/1 -> Add26/2
  Constant74/1 -> Add27/1
  Product58/1 -> Add27/2
  Constant73/1 -> Product59/1
  Add27/1 -> Product59/2
  Add26/1 -> Add28/1
  Product59/1 -> Add28/2
  Product57/1 -> Product60/1
  Add28/1 -> Product60/2
  Product60/1 -> Product61/1
  [DEN2] -> Product61/2
  Product61/1 -> [K011]
  Constant77/1 -> Product62/1
  P_15/1 -> Product62/2
  Constant76/1 -> Add29/1
  Product62/1 -> Add29/2
  Add29/1 -> Product63/1
  [DEN2] -> Product63/2
  Product63/1 -> [K012]
  Constant79/1 -> Product64/1
  P_16/1 -> Product64/2
  Constant78/1 -> Add30/1
  Product64/1 -> Add30/2
  Constant81/1 -> Product65/1
  P_17/1 -> Product65/2
  Constant80/1 -> Add31/1
  Product65/1 -> Add31/2
  X_e_6/1 -> Product66/1
  Add31/1 -> Product66/2
  Add30/1 -> Add32/1
  Product66/1 -> Add32/2
  Constant82/1 -> Product67/1
  Add32/1 -> Product67/2
  Product67/1 -> Product68/1
  [DEN2] -> Product68/2
  Product68/1 -> [K013]
  Constant87/1 -> Product69/1
  P_18/1 -> Product69/2
  Constant86/1 -> Add33/1
  Product69/1 -> Add33/2
  Constant89/1 -> Product70/1
  P_19/1 -> Product70/2
  Constant88/1 -> Add34/1
  Product70/1 -> Add34/2
  X_e_7/1 -> Product71/1
  Add34/1 -> Product71/2
  Constant85/1 -> Add35/1
  L_s1_6/1 -> Add35/2
  Constant84/1 -> Product72/2
  Add35/1 -> Product72/3
  Constant83/1 -> Product72/1
  Product71/1 -> Product73/1
  Constant90/1 -> Product73/2
  Product73/1 -> Add36/2
  Add33/1 -> Add36/1
  Product72/1 -> Product74/1
  Add36/1 -> Product74/2
  Product74/1 -> Product75/1
  [DEN2] -> Product75/2
  Product75/1 -> [K014]
  Constant93/1 -> Product76/1
  P_20/1 -> Product76/2
  Constant92/1 -> Add37/1
  Product76/1 -> Add37/2
  Constant95/1 -> Product77/1
  P_21/1 -> Product77/2
  Constant94/1 -> Add38/1
  Product77/1 -> Add38/2
  X_e_8/1 -> Product78/1
  Add38/1 -> Product78/2
  Product78/1 -> Product79/1
  Constant96/1 -> Product79/2
  Product79/1 -> Add39/2
  Add37/1 -> Add39/1
  Constant91/1 -> Product81/1
  DENS_b_2/1 -> Product81/2
  Add39/1 -> Product81/3
  Product81/1 -> Product82/1
  [DEN2] -> Product82/2
  Product82/1 -> [K015]
  Constant99/1 -> Add41/1
  L_s1_7/1 -> Add41/2
  X_e_9/1 -> Product83/1
  Constant101/1 -> Product83/2
  Product83/1 -> Product84/1
  Constant102/1 -> Product84/2
  Constant100/1 -> Add42/1
  Product84/1 -> Add42/2
  Constant103/1 -> Product85/1
  Constant98/1 -> Product85/2
  Add41/1 -> Product85/3
  Product85/1 -> Product86/1
  Add42/1 -> Product86/2
  Product86/1 -> Product87/1
  [DEN2] -> Product87/2
  Product87/1 -> [K016]
  Constant104/1 -> Product88/1
  Constant105/1 -> Product88/2
  Product88/1 -> [K017]
  Constant106/1 -> Product89/1
  Constant107/1 -> Product89/2
  W_fi/1 -> Product90/1
  Product89/1 -> Product90/2
  Product90/1 -> [K018]
  Constant108/1 -> Add43/1
  X_e_10/1 -> Add43/2
  Constant109/1 -> Product91/1
  Constant110/1 -> Product91/2
  Add43/1 -> Product92/1
  Product91/1 -> Product92/2
  Product92/1 -> [K019]
  Constant112/1 -> Product93/1
  Constant113/1 -> Product93/2
  Constant111/1 -> Product94/1
  W1/1 -> Product94/2
  Product94/1 -> Product95/1
  Product93/1 -> Product95/2
  Product95/1 -> [K020]
  Constant115/1 -> Product97/1
  Constant116/1 -> Product97/2
  [L_dw] -> Product97/3
  W_fi_1/1 -> Product96/1
  Product96/1 -> Product98/1
  Product97/1 -> Product98/2
  Product98/1 -> [K021]
  Constant118/1 -> Add44/1
  X_e_11/1 -> Add44/2
  Constant120/1 -> Product99/1
  P_22/1 -> Product99/2
  Constant119/1 -> Add45/1
  Product99/1 -> Add45/2
  Constant121/1 -> Product100/1
  Constant122/1 -> Product100/2
  Product100/1 -> Product102/2
  Add44/1 -> Product101/1
  Add45/1 -> Product101/2
  Product101/1 -> Product102/1
  Product102/1 -> [K022]
  Constant124/1 -> Product103/1
  Constant125/1 -> Product103/2
  Constant127/1 -> Product104/1
  W1_1/1 -> Product104/2
  T_d_3/1 -> Product104/3
  Product104/1 -> Product105/1
  Product103/1 -> Product105/2
  Product105/1 -> [K023]
  Constant134/1 -> Product106/1
  [T_dw] -> Product106/2
  Constant128/1 -> Product106/3
  Constant129/1 -> Product106/4
  Constant130/1 -> Product107/1
  Constant131/1 -> Product107/2
  [L_dw] -> Product107/3
  Product106/1 -> Product108/1
  Product107/1 -> Product108/2
  Product108/1 -> [K024]
  Constant137/1 -> Product109/1
  [L_dw] -> Product109/2
  Product109/1 -> Add46/2
  Constant136/1 -> Add46/1
  Constant135/1 -> Product110/1
  Add46/1 -> Product110/2
  X_e_12/1 -> Product111/1
  Product110/1 -> Product111/2
  Product111/1 -> [K025]
  Constant143/1 -> Product112/1
  Product112/1 -> Add47/2
  Constant142/1 -> Add47/1
  Constant141/1 -> Product113/1
  Add47/1 -> Product113/2
  [C_l] -> Product114/2
  Constant139/1 -> Product114/1
  P_23/1 -> Product114/3
  Product114/1 -> Product115/1
  Product113/1 -> Product115/2
  Product115/1 -> [K026]
  Constant146/1 -> Product116/1
  P_24/1 -> Product116/2
  Constant145/1 -> Add48/1
  Product116/1 -> Add48/2
  Add48/1 -> Product117/1
  Constant147/1 -> Product117/2
  Constant151/1 -> Product118/1
  Constant149/1 -> Add49/1
  Product118/1 -> Add49/2
  Constant148/1 -> Product119/1
  Add49/1 -> Product119/2
  Product117/1 -> Product120/1
  Product119/1 -> Product120/2
  Product120/1 -> [K027]
  [K019] -> Product121/1
  W1_2/1 -> Product121/2
  [K018] -> Add50/1
  Product121/1 -> Add50/2
  [K020] -> Add50/3
  Add50/1 -> [P1]
  [K05] -> Add51/1
  [K010] -> Add51/2
  [K019] -> Product122/1
  Add51/1 -> Product122/2
  Product122/1 -> [P2]
  [K019] -> Product124/2
  Product124/1 -> [P3]
  [K019] -> Product126/2
  Product126/1 -> [P4]
  [K022] -> Product127/1
  W1_4/1 -> Product127/2
  [K024] -> Product128/1
  [P1] -> Product128/2
  [K021] -> Add52/1
  Product127/1 -> Add52/2
  [K023] -> Add52/3
  Product128/1 -> Add52/4
  Add52/1 -> P5/1
  [K05] -> Add53/1
  [K010] -> Add53/2
  [K024] -> Product26/1
  [P2] -> Product26/2
  Add53/1 -> Product24/2
  Product24/1 -> Add56/1
  Product26/1 -> Add56/2
  Add56/1 -> P6/1
  [K024] -> Product129/1
  [P3] -> Product129/2
  [K017] -> Product131/1
  [K03] -> Product131/2
  [K09] -> Product130/1
  [K01] -> Product130/2
  [K017] -> Product125/1
  [K04] -> Product125/2
  [K09] -> Product132/1
  [K02] -> Product132/2
  Product125/1 -> Add57/1
  Product132/1 -> Add57/2
  Add57/1 -> Product126/1
  [K017] -> Product123/1
  [K03] -> Product123/2
  [K09] -> Product133/1
  [K01] -> Product133/2
  Product123/1 -> Add58/1
  Product133/1 -> Add58/2
  Add58/1 -> Product124/1
  Product131/1 -> Add59/1
  Product130/1 -> Add59/2
  [K022] -> Product134/1
  Add59/1 -> Product134/2
  Product134/1 -> Add60/1
  Product129/1 -> Add60/2
  Add60/1 -> P7/1
  [K017] -> Product135/1
  [K04] -> Product135/2
  [K09] -> Product136/1
  [K02] -> Product136/2
  Product135/1 -> Add61/1
  Product136/1 -> Add61/2
  [K024] -> Product137/1
  [P4] -> Product137/2
  Add61/1 -> Product138/1
  [K022] -> Product138/2
  Product138/1 -> Add62/1
  Product137/1 -> Add62/2
  Add62/1 -> P8/1
  [K025] -> Product139/1
  W1_5/1 -> Product139/2
  [K027] -> Product140/1
  [P1] -> Product140/2
  Product139/1 -> Add63/1
  [K026] -> Add63/2
  Product140/1 -> Add63/3
  [K017] -> Product141/1
  [K03] -> Product141/2
  [K09] -> Product142/1
  [K01] -> Product142/2
  Product141/1 -> Add64/1
  Product142/1 -> Add64/2
  Add64/1 -> Product143/1
  [K025] -> Product143/2
  [K027] -> Product144/1
  [P3] -> Product144/2
  Constant152/1 -> Add65/1
  Product143/1 -> Add65/2
  Product144/1 -> Add65/3
  Add63/1 -> Product145/1
  Add65/1 -> Product145/2
  Product145/1 -> P9/1
  [K010] -> Add66/2
  [K05] -> Add66/1
  [K025] -> Product146/1
  Add66/1 -> Product146/2
  [K027] -> Product147/1
  [P2] -> Product147/2
  Product146/1 -> Add67/1
  Product147/1 -> Add67/2
  [K017] -> Product148/1
  [K03] -> Product148/2
  [K09] -> Product149/1
  [K01] -> Product149/2
  Product148/1 -> Add68/1
  Product149/1 -> Add68/2
  Add68/1 -> Product150/1
  [K025] -> Product150/2
  [K027] -> Product151/1
  [P3] -> Product151/2
  Constant153/1 -> Add69/1
  Product150/1 -> Add69/2
  Product151/1 -> Add69/3
  Add67/1 -> Product152/1
  Add69/1 -> Product152/2
  Product152/1 -> P10/1
  [K04] -> Product153/2
  [K017] -> Product153/1
  [K09] -> Product154/1
  [K02] -> Product154/2
  Product153/1 -> Add70/1
  Product154/1 -> Add70/2
  Add70/1 -> Product155/1
  [K025] -> Product155/2
  [K027] -> Product156/1
  [P4] -> Product156/2
  Product155/1 -> Add71/1
  Product156/1 -> Add71/2
  [K017] -> Product157/1
  [K03] -> Product157/2
  [K09] -> Product158/1
  [K01] -> Product158/2
  Product157/1 -> Add72/1
  Product158/1 -> Add72/2
  Add72/1 -> Product159/1
  [K025] -> Product159/2
  [K027] -> Product160/1
  [P3] -> Product160/2
  Constant154/1 -> Add73/1
  Product159/1 -> Add73/2
  Product160/1 -> Add73/3
  Add71/1 -> Product161/1
  Add73/1 -> Product161/2
  Product161/1 -> P11/1
  [K07] -> Product162/1
  W1_6/1 -> Product162/2
  [K05] -> Product163/1
  [K07] -> Product163/2
  [K06] -> Add74/1
  Product162/1 -> Add74/2
  Constant155/1 -> Add75/1
  Product163/1 -> Add75/2
  Add74/1 -> Product164/1
  Add75/1 -> Product164/2
  Product164/1 -> P12/1
  [K05] -> Product165/1
  [K07] -> Product165/2
  Product165/1 -> Add76/2
  Constant156/1 -> Add76/1
  [K08] -> Product166/1
  Add76/1 -> Product166/2
  Product166/1 -> P13/1
  [K013] -> Add77/1
  [K012] -> Add77/2
  Add77/1 -> Product167/1
  W1_3/1 -> Product167/2
  [K011] -> Add78/1
  Product167/1 -> Add78/2
  [K02] -> Product168/1
  [K09] -> Product168/2
  [K013] -> Product168/3
  [K014] -> Product169/1
  [K02] -> Product169/2
  Product168/1 -> Add79/1
  Product169/1 -> Add79/2
  Constant157/1 -> Add80/1
  Add79/1 -> Add80/2
  Add78/1 -> Product170/1
  Add80/1 -> Product170/2
  Product170/1 -> P14/1
  [K05] -> Add81/1
  [K010] -> Add81/2
  [K013] -> Product172/2
  Add81/1 -> Product172/1
  [K012] -> Product171/1
  [K05] -> Product171/2
  Product171/1 -> Add82/1
  Product172/1 -> Add82/2
  [K015] -> Add82/3
  [K02] -> Product173/1
  [K09] -> Product173/2
  [K013] -> Product173/3
  [K014] -> Product174/1
  [K02] -> Product174/2
  Product173/1 -> Add83/1
  Product174/1 -> Add83/2
  Constant158/1 -> Add84/1
  Add83/1 -> Add84/2
  Add82/1 -> Product175/1
  Add84/1 -> Product175/2
  Product175/1 -> P15/1
  [K02] -> Product176/1
  [K09] -> Product176/2
  [K013] -> Product176/3
  [K014] -> Product177/1
  [K02] -> Product177/2
  Product176/1 -> Add85/1
  Product177/1 -> Add85/2
  Constant159/1 -> Add86/1
  Add85/1 -> Add86/2
  [K09] -> Product178/2
  [K01] -> Product178/1
  [K013] -> Product178/3
  [K014] -> Product179/1
  [K01] -> Product179/2
  Product178/1 -> Add87/1
  Product179/1 -> Add87/2
  [K016] -> Add87/3
  Add87/1 -> Product180/1
  Add86/1 -> Product180/2
  Product180/1 -> P16/1
  T_fi/1 -> Product96/2
  L_dw/1 -> [L_dw]
  [L_dw] -> Product100/3
  [L_dw] -> Product103/3
  T_dw/1 -> [T_dw]
  C_l/1 -> [C_l]
  [L_dw] -> Product112/2
  [L_dw] -> Product118/2
  Add7/1 -> Math Function/1
  Product19/1 -> Product16/1
  Constant24/1 -> Product16/2
  Product16/1 -> Product25/1
  Add11/1 -> Math Function1/1
  Add15/1 -> Math Function2/1
  Add19/1 -> Math Function3/1
  [K022] -> Product24/1

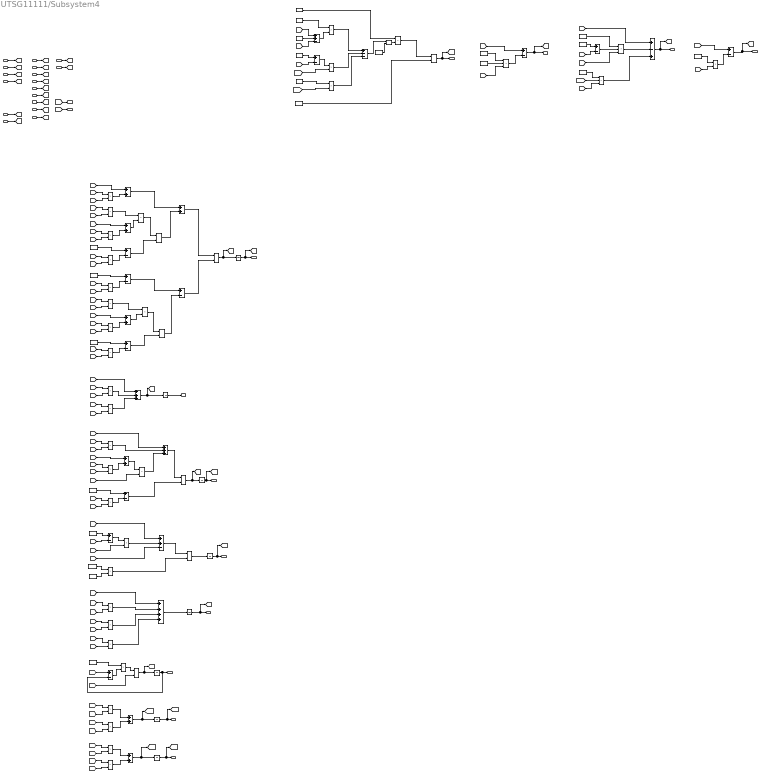
== system UTSG11111/Subsystem4 ==
  note: W1
  note: W4
  note: W3
  note: W2
  note: DENS_r
  note: DENS_b
  note: T_d
  note: T_dw
  note: L_dw
  note: X_e
  note: P
  note: AUX1 DLs1
  K01 : Inport
  K02 : Inport  Port=2
  K03 : Inport  Port=3
  K04 : Inport  Port=4
  P5 : Inport  Port=5
  P6 : Inport  Port=6
  P7 : Inport  Port=7
  P8 : Inport  Port=8
  P9 : Inport  Port=9
  P10 : Inport  Port=10
  P11 : Inport  Port=11
  P12 : Inport  Port=12
  P13 : Inport  Port=13
  P14 : Inport  Port=14
  P15 : Inport  Port=15
  P16 : Inport  Port=16
  W_fi : Inport  Port=17
  Add10 : Sum  Inputs=+++
  Add{2,4..5,7,11,18..19} (7 alike) : Sum
  Add{3,6,8..9,12,14,17,21,23..24,26} (11 alike) : Sum  Inputs=+-
  Add13 : Sum  Inputs=+++
  Add15 : Sum  Inputs=++-
  Add16 : Sum  Inputs=++++
  Add20 : Sum  Inputs=++-
  Add22 : Sum  Inputs=+--
  Add25 : Sum  Inputs=+-+
  Constant1 : Constant  Value=DENS_dw
  Constant10 : Constant  Value=DENS_d
  Constant11 : Constant  Value=L_d
  Constant12 : Constant  Value=L
  Constant13 : Constant  Value=L_r
  Constant14 : Constant  Value=12
  Constant15 : Constant  Value=DENS_s
  Constant16 : Constant  Value=A_fs
  Constant17 : Constant  Value=A_fs
  Constant18 : Constant  Value=L
  Constant19 : Constant  Value=A_fs
  Constant{2..6} (5 alike) : Constant
  Constant20 : Constant  Value=V_r
  Constant21 : Constant  Value=0.5
  Constant7 : Constant  Value=A_dw
  Constant8 : Constant  Value=M_d
  Constant9 : Constant  Value=C_1
  Math Function : Math  Operator=pow  SaturateOnIntegerOverflow=on
  Product{2..6,8..12,15..20,22..23,25..28,30..37,42} (31 alike) : Product
  Product{7,13..14,21,24,29,38} (7 alike) : Product  Inputs=*/
  Product39 : Product  Inputs=3
  Product40 : Product  Inputs=3
  Product41 : Product  Inputs=3
  dDENS_b/dt : Integrator  InitialCondition=13.614
  dDENS_r/dt1 : Integrator  InitialCondition=7.94
  dL_dw/dt : Integrator  InitialCondition=9.63
  dL_s1/dt : Integrator  InitialCondition=3.4517
  dP/dt : Integrator  InitialCondition=849.7
  dT_d/dt : Integrator  InitialCondition=504.7
  dT_dw/dt : Integrator  InitialCondition=504.7
  dX_e/dt : Integrator  InitialCondition=0.2
  L_s1 : Outport
  P : Outport  Port=2
  X_e : Outport  Port=3
  L_dw : Outport  Port=4
  T_dw : Outport  Port=5
  T_d : Outport  Port=6
  DENS_b : Outport  Port=7
  DENS_r : Outport  Port=8
  W1 : Outport  Port=9
  W2 : Outport  Port=10
  W3 : Outport  Port=11
  W4 : Outport  Port=12
  AUX1 : Outport  Port=13
  AUX6 : Outport  Port=14
  wires:
  K01/1 -> [K01]
  K02/1 -> [K02]
  K03/1 -> [K03]
  K04/1 -> [K04]
  P5/1 -> [P5]
  P6/1 -> [P6]
  P7/1 -> [P7]
  P8/1 -> [P8]
  P9/1 -> [P9]
  P10/1 -> [P10]
  P11/1 -> [P11]
  P12/1 -> [P12]
  P13/1 -> [P13]
  P14/1 -> [P14]
  P15/1 -> [P15]
  P16/1 -> [P16]
  [P13] -> Product2/1
  [P9] -> Product2/2
  [P16] -> Product3/1
  [P9] -> Product3/2
  [P14] -> Add2/1
  Product3/1 -> Add2/2
  [P13] -> Product4/1
  [P11] -> Product4/2
  Add2/1 -> Product5/2
  Product4/1 -> Product5/1
  [P16] -> Product6/1
  [P11] -> Product6/2
  Constant2/1 -> Add3/1
  Product6/1 -> Add3/2
  Product5/1 -> Product7/1
  Add3/1 -> Product7/2
  [P12] -> Add4/1
  Product2/1 -> Add4/2
  Add4/1 -> Add5/1
  Product7/1 -> Add5/2
  [P10] -> Product8/1
  [P13] -> Product8/2
  Constant3/1 -> Add6/1
  Product8/1 -> Add6/2
  [P16] -> Product9/1
  [P10] -> Product9/2
  [P15] -> Add7/1
  Product9/1 -> Add7/2
  [P13] -> Product10/1
  [P11] -> Product10/2
  Product10/1 -> Product11/1
  Add7/1 -> Product11/2
  [P16] -> Product12/1
  [P11] -> Product12/2
  Constant4/1 -> Add8/1
  Product12/1 -> Add8/2
  Product11/1 -> Product13/1
  Add8/1 -> Product13/2
  Add6/1 -> Add9/1
  Product13/1 -> Add9/2
  Add5/1 -> Product14/1
  Add9/1 -> Product14/2
  Product14/1 -> [AUX1], dL_s1/dt/1
  dL_s1/dt/1 -> [L_s1], L_s1/1
  [P10] -> Product15/1
  [AUX1] -> Product15/2
  [P11] -> Product16/1
  [AUX3] -> Product16/2
  [P9] -> Add10/1
  Product15/1 -> Add10/2
  Product16/1 -> Add10/3
  Add10/1 -> [AUX2], dP/dt/1
  dP/dt/1 -> P/1
  [P16] -> Product17/1
  [P9] -> Product17/2
  [P10] -> Product18/2
  [P16] -> Product18/1
  [P15] -> Add11/1
  Product18/1 -> Add11/2
  Add11/1 -> Product19/1
  [AUX1] -> Product19/2
  [P16] -> Product20/1
  [P11] -> Product20/2
  Constant5/1 -> Add12/1
  Product20/1 -> Add12/2
  [P14] -> Add13/1
  Product17/1 -> Add13/2
  Product19/1 -> Add13/3
  Add13/1 -> Product21/1
  Add12/1 -> Product21/2
  Product21/1 -> [AUX3], dX_e/dt/1
  dX_e/dt/1 -> [X_e], X_e/1
  W_fi/1 -> [W_fi]
  Constant1/1 -> Product22/1
  Constant7/1 -> Product22/2
  Constant6/1 -> Add14/1
  [X_e] -> Add14/2
  Add14/1 -> Product23/1
  [W4] -> Product23/2
  [W_fi] -> Add15/1
  Product23/1 -> Add15/2
  [W1] -> Add15/3
  Add15/1 -> Product24/1
  Product22/1 -> Product24/2
  Product24/1 -> dL_dw/dt/1
  dL_dw/dt/1 -> [L_dw], L_dw/1
  [P6] -> Product25/1
  [AUX1] -> Product25/2
  [P7] -> Product26/1
  [AUX2] -> Product26/2
  [AUX3] -> Product27/2
  [P8] -> Product27/1
  [P5] -> Add16/1
  Product25/1 -> Add16/2
  Product26/1 -> Add16/3
  Product27/1 -> Add16/4
  Add16/1 -> dT_dw/dt/1
  dT_dw/dt/1 -> [T_dw], T_dw/1
  [T_dw] -> Add17/1
  dT_d/dt/1 -> T_d/1, Add17/2
  Constant8/1 -> Product28/1
  Add17/1 -> Product28/2
  Product28/1 -> Product29/1
  [W1] -> Product29/2
  Product29/1 -> [AUX6], dT_d/dt/1
  [K01] -> Product30/1
  [AUX2] -> Product30/2
  [K02] -> Product31/1
  [AUX3] -> Product31/2
  Product30/1 -> Add18/1
  Product31/1 -> Add18/2
  Add18/1 -> [AUX7], dDENS_b/dt/1
  dDENS_b/dt/1 -> [DENS_b], DENS_b/1
  [K04] -> Product33/1
  [AUX3] -> Product33/2
  [K03] -> Product32/1
  [AUX2] -> Product32/2
  Product32/1 -> Add19/1
  Product33/1 -> Add19/2
  Add19/1 -> [AUX8], dDENS_r/dt1/1
  dDENS_r/dt1/1 -> [DENS_r], DENS_r/1
  [L_dw] -> Add20/1
  Constant11/1 -> Add20/2
  [L_s1] -> Add20/3
  Constant12/1 -> Add21/1
  [L_s1] -> Add21/2
  Constant10/1 -> Product34/1
  Add20/1 -> Product34/2
  Add21/1 -> Product35/1
  [DENS_b] -> Product35/2
  Constant13/1 -> Product36/1
  [DENS_r] -> Product36/2
  Product34/1 -> Add22/1
  Product35/1 -> Add22/2
  Product36/1 -> Add22/3
  Constant9/1 -> Product37/1
  Add22/1 -> Math Function/1
  Constant14/1 -> Product38/2
  Product38/1 -> W1/1, [W1]
  Constant15/1 -> Product39/1
  Constant16/1 -> Product39/2
  [AUX1] -> Product39/3
  [W1] -> Add23/1
  Product39/1 -> Add23/2
  Add23/1 -> [W2], W2/1
  Constant18/1 -> Add24/1
  [L_s1] -> Add24/2
  Constant17/1 -> Product40/1
  Add24/1 -> Product40/2
  [AUX7] -> Product40/3
  Constant19/1 -> Product41/1
  [DENS_b] -> Product41/2
  [AUX1] -> Product41/3
  [W2] -> Add25/1
  Product40/1 -> Add25/2
  Product41/1 -> Add25/3
  Add25/1 -> [W3], W3/1
  Constant20/1 -> Product42/1
  [AUX8] -> Product42/2
  [W3] -> Add26/1
  Product42/1 -> Add26/2
  Add26/1 -> [W4], W4/1
  [AUX1] -> AUX1/1
  [AUX6] -> AUX6/1
  Constant21/1 -> Math Function/2
  Math Function/1 -> Product37/2
  Product37/1 -> Product38/1
